simulink model "integrator_matrix_test"  (Simulink 8.4)
settings: Solver=ode45  StartTime=0.0  StopTime=10.0  RelTol=1e-3
settings Model: Creator=arnaud  LastModifiedBy=arnaud
settings DataIOCC: SaveFormat=Structure

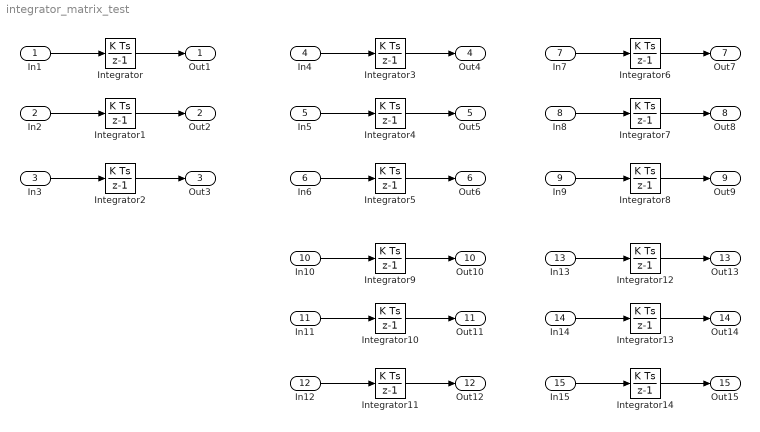
== system integrator_matrix_test ==
  In1 : Inport  OutDataTypeStr=double  PortDimensions=[2 3]
  In2 : Inport  Port=2  OutDataTypeStr=int8  PortDimensions=[2 3]
  In3 : Inport  Port=3  OutDataTypeStr=boolean  PortDimensions=[2 3]
  In4 : Inport  Port=4  OutDataTypeStr=double  PortDimensions=[2 3]
  In5 : Inport  Port=5  OutDataTypeStr=int8  PortDimensions=[2 3]
  In6 : Inport  Port=6  OutDataTypeStr=boolean  PortDimensions=[2 3]
  In7 : Inport  Port=7  OutDataTypeStr=double  PortDimensions=1
  In8 : Inport  Port=8  OutDataTypeStr=int8  PortDimensions=1
  In9 : Inport  Port=9  OutDataTypeStr=boolean  PortDimensions=1
  In10 : Inport  Port=10  OutDataTypeStr=double  PortDimensions=[2 3]
  In11 : Inport  Port=11  OutDataTypeStr=int8  PortDimensions=[2 3]
  In12 : Inport  Port=12  OutDataTypeStr=boolean  PortDimensions=[2 3]
  In13 : Inport  Port=13  OutDataTypeStr=double  PortDimensions=1
  In14 : Inport  Port=14  OutDataTypeStr=int8  PortDimensions=1
  In15 : Inport  Port=15  OutDataTypeStr=boolean  PortDimensions=1
  Integrator : DiscreteIntegrator  SampleTime=1.0  mask(DiscretizedDiscreteIntegrator){}
      mask init:
      | %zoh
  Integrator1 : DiscreteIntegrator  SampleTime=1.0  mask(DiscretizedDiscreteIntegrator){}
      mask init:
      | %zoh
  Integrator10 : DiscreteIntegrator  gainval=[1.0 20 3.0; 5 4.0 6]  InitialCondition=[0.0 -0 -3.0; 6 8.0 -2]  SampleTime=1.0  mask(DiscretizedDiscreteIntegrator){}
      mask init:
      | %zoh
  Integrator11 : DiscreteIntegrator  gainval=[1.0 20 3.0; 5 4.0 6]  InitialCondition=[0.0 -0 -3.0; 6 8.0 -2]  SampleTime=1.0  mask(DiscretizedDiscreteIntegrator){}
      mask init:
      | %zoh
  Integrator12 : DiscreteIntegrator  gainval=[1.0 20 3.0; 5 4.0 6]  InitialCondition=[0.0 -0 -3.0; 6 8.0 -2]  SampleTime=1.0  mask(DiscretizedDiscreteIntegrator){}
      mask init:
      | %zoh
  Integrator13 : DiscreteIntegrator  gainval=[1.0 20 3.0; 5 4.0 6]  InitialCondition=[0.0 -0 -3.0; 6 8.0 -2]  SampleTime=1.0  mask(DiscretizedDiscreteIntegrator){}
      mask init:
      | %zoh
  Integrator14 : DiscreteIntegrator  gainval=[1.0 20 3.0; 5 4.0 6]  InitialCondition=[0.0 -0 -3.0; 6 8.0 -2]  SampleTime=1.0  mask(DiscretizedDiscreteIntegrator){}
      mask init:
      | %zoh
  Integrator2 : DiscreteIntegrator  SampleTime=1.0  mask(DiscretizedDiscreteIntegrator){}
      mask init:
      | %zoh
  Integrator3 : DiscreteIntegrator  gainval=[1.0 20 3.0; 5 4.0 6]  SampleTime=1.0  mask(DiscretizedDiscreteIntegrator){}
      mask init:
      | %zoh
  Integrator4 : DiscreteIntegrator  gainval=[1.0 20 3.0; 5 4.0 6]  SampleTime=1.0  mask(DiscretizedDiscreteIntegrator){}
      mask init:
      | %zoh
  Integrator5 : DiscreteIntegrator  gainval=[1.0 20 3.0; 5 4.0 6]  SampleTime=1.0  mask(DiscretizedDiscreteIntegrator){}
      mask init:
      | %zoh
  Integrator6 : DiscreteIntegrator  gainval=[1.0 20 3.0; 5 4.0 6]  SampleTime=1.0  mask(DiscretizedDiscreteIntegrator){}
      mask init:
      | %zoh
  Integrator7 : DiscreteIntegrator  gainval=[1.0 20 3.0; 5 4.0 6]  SampleTime=1.0  mask(DiscretizedDiscreteIntegrator){}
      mask init:
      | %zoh
  Integrator8 : DiscreteIntegrator  gainval=[1.0 20 3.0; 5 4.0 6]  SampleTime=1.0  mask(DiscretizedDiscreteIntegrator){}
      mask init:
      | %zoh
  Integrator9 : DiscreteIntegrator  gainval=[1.0 20 3.0; 5 4.0 6]  InitialCondition=[0.0 -0 -3.0; 6 8.0 -2]  SampleTime=1.0  mask(DiscretizedDiscreteIntegrator){}
      mask init:
      | %zoh
  Out1 : Outport
  Out2 : Outport  Port=2
  Out3 : Outport  Port=3
  Out4 : Outport  Port=4
  Out5 : Outport  Port=5
  Out6 : Outport  Port=6
  Out7 : Outport  Port=7
  Out8 : Outport  Port=8
  Out9 : Outport  Port=9
  Out10 : Outport  Port=10
  Out11 : Outport  Port=11
  Out12 : Outport  Port=12
  Out13 : Outport  Port=13
  Out14 : Outport  Port=14
  Out15 : Outport  Port=15
  wires:
  In1/1 -> Integrator/1
  Integrator/1 -> Out1/1
  In2/1 -> Integrator1/1
  Integrator1/1 -> Out2/1
  In3/1 -> Integrator2/1
  Integrator2/1 -> Out3/1
  In4/1 -> Integrator3/1
  Integrator3/1 -> Out4/1
  In5/1 -> Integrator4/1
  Integrator4/1 -> Out5/1
  In6/1 -> Integrator5/1
  Integrator5/1 -> Out6/1
  In7/1 -> Integrator6/1
  Integrator6/1 -> Out7/1
  In8/1 -> Integrator7/1
  Integrator7/1 -> Out8/1
  In9/1 -> Integrator8/1
  Integrator8/1 -> Out9/1
  In10/1 -> Integrator9/1
  Integrator9/1 -> Out10/1
  In11/1 -> Integrator10/1
  Integrator10/1 -> Out11/1
  In12/1 -> Integrator11/1
  Integrator11/1 -> Out12/1
  In13/1 -> Integrator12/1
  Integrator12/1 -> Out13/1
  In14/1 -> Integrator13/1
  Integrator13/1 -> Out14/1
  In15/1 -> Integrator14/1
  Integrator14/1 -> Out15/1
